simulink model "simproject2"  (R2022b)
settings: Solver=VariableStepAuto  StartTime=0.0  StopTime=Tsim  RelTol=1e-3
values from neighbouring files (symbols this model uses):
  Aroad = 5    [project2.m]
  Caf = 60000    [project2.m]
  Car = 60000    [project2.m]
  Iz = 2000    [project2.m]
  lambdaRoad = 100    [project2.m]
  lf = 1.1    [project2.m]
  lr = 1.3    [project2.m]
  m = 1050    [project2.m]
  Vx = 100/3.6    (= 27.7777777778)    [project2.m]
settings Model: Creator=Forough  LastModifiedBy=Forough

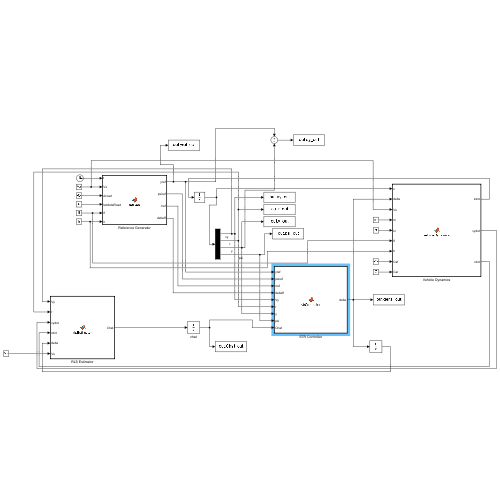
[thumbnail: Simulink's stored preview of the top-level diagram]
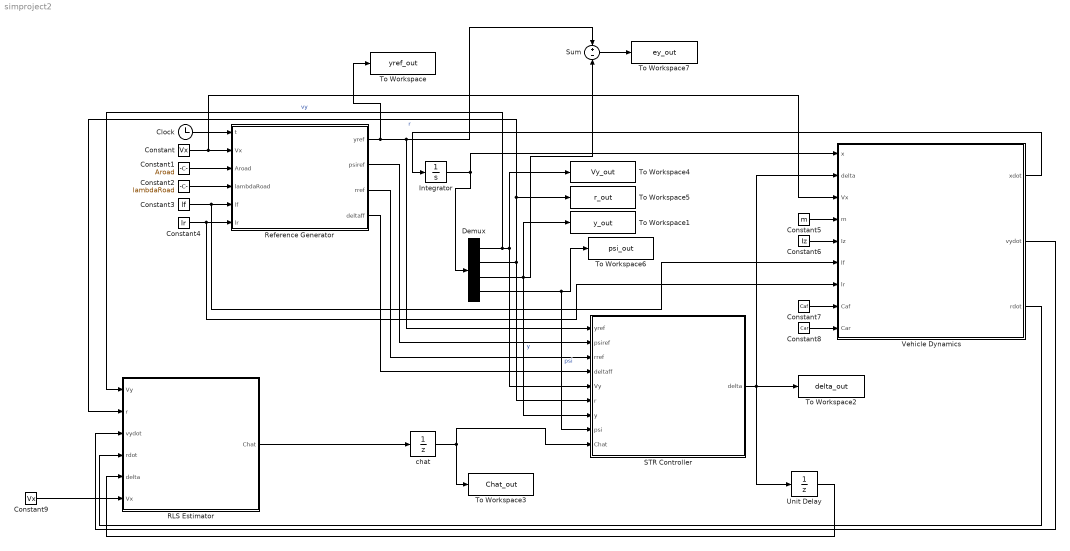
== system simproject2 ==
  Clock : Clock
  Constant : Constant  Value=Vx
  Constant1 : Constant  Value=Aroad
  Constant2 : Constant  Value=lambdaRoad
  Constant3 : Constant  Value=lf
  Constant4 : Constant  Value=lr
  Constant5 : Constant  Value=m
  Constant6 : Constant  Value=Iz
  Constant7 : Constant  Value=Caf
  Constant8 : Constant  Value=Car
  Constant9 : Constant  Value=Vx
  Demux : Demux
  Integrator : Integrator  InitialCondition=[0;0;0;0]
  RLS Estimator : MATLAB Function  TreatAsAtomicUnit=on
  Reference Generator : MATLAB Function  TreatAsAtomicUnit=on
  STR Controller : MATLAB Function  TreatAsAtomicUnit=on
  Sum : Sum  Inputs=+-
  To Workspace : ToWorkspace  VariableName=yref_out  SaveFormat=Timeseries  SampleTime=-1
  To Workspace1 : ToWorkspace  VariableName=y_out  SaveFormat=Timeseries  SampleTime=-1
  To Workspace2 : ToWorkspace  VariableName=delta_out  SaveFormat=Timeseries  SampleTime=-1
  To Workspace3 : ToWorkspace  VariableName=Chat_out  SaveFormat=Timeseries  SampleTime=-1
  To Workspace4 : ToWorkspace  VariableName=Vy_out  SaveFormat=Timeseries  SampleTime=-1
  To Workspace5 : ToWorkspace  VariableName=r_out  SaveFormat=Timeseries  SampleTime=-1
  To Workspace6 : ToWorkspace  VariableName=psi_out  SaveFormat=Timeseries  SampleTime=-1
  To Workspace7 : ToWorkspace  VariableName=ey_out  SaveFormat=Timeseries  SampleTime=-1
  Unit Delay : UnitDelay  SampleTime=0.001  HasFrameUpgradeWarning=on
  Vehicle Dynamics : MATLAB Function  TreatAsAtomicUnit=on
  chat : UnitDelay  InitialCondition=60000  SampleTime=0.001  HasFrameUpgradeWarning=on
  wires:
  Clock/1 -> Reference Generator/1(t)
  Integrator/1 -> Demux/1, Vehicle Dynamics/1(x)
  Vehicle Dynamics/1(xdot) -> Integrator/1
  Constant/1 -> Vehicle Dynamics/3(Vx), Reference Generator/2(Vx)
  Constant1/1 -> Reference Generator/3(Aroad)
  Constant2/1 -> Reference Generator/4(lambdaRoad)
  Constant3/1 -> Vehicle Dynamics/6(lf), Reference Generator/5(lf)
  Constant4/1 -> Vehicle Dynamics/7(lr), Reference Generator/6(lr)
  Reference Generator/1(yref) -> To Workspace/1, Sum/1, STR Controller/1(yref)
  Reference Generator/2(psiref) -> STR Controller/2(psiref)
  Reference Generator/3(rref) -> STR Controller/3(rref)
  Reference Generator/4(deltaff) -> STR Controller/4(deltaff)
  Demux/1 -> RLS Estimator/1(Vy), To Workspace4/1, STR Controller/5(Vy)  "vy"
  Demux/2 -> To Workspace5/1, RLS Estimator/2(r), STR Controller/6(r)  "r"
  Demux/3 -> Sum/2, To Workspace1/1, STR Controller/7(y)  "y"
  Demux/4 -> To Workspace6/1, STR Controller/8(psi)  "psi"
  RLS Estimator/1(Chat) -> chat/1
  STR Controller/1(delta) -> Unit Delay/1, To Workspace2/1, Vehicle Dynamics/2(delta)
  Unit Delay/1 -> RLS Estimator/5(delta)
  Vehicle Dynamics/2(vydot) -> RLS Estimator/3(vydot)
  Vehicle Dynamics/3(rdot) -> RLS Estimator/4(rdot)
  Constant5/1 -> Vehicle Dynamics/4(m)
  Constant6/1 -> Vehicle Dynamics/5(Iz)
  Constant7/1 -> Vehicle Dynamics/8(Caf)
  Constant8/1 -> Vehicle Dynamics/9(Car)
  chat/1 -> To Workspace3/1, STR Controller/9(Chat)
  Sum/1 -> To Workspace7/1
  Constant9/1 -> RLS Estimator/6(Vx)

== matlab function simproject2/Vehicle Dynamics ==
  data: x input; xdot output; delta input; Vx input; m input; Iz input; lf input; lr input; Caf input; Car input; vydot output; rdot output
function [xdot, vydot, rdot] = vehicleDynamics(x, delta, Vx, m, Iz, lf, lr, Caf, Car)

% States
Vy  = x(1);
r   = x(2);
y   = x(3);
psi = x(4);

% Lateral velocity dynamics
vydot = ...
    - ((2*Caf + 2*Car)/(m*Vx))*Vy ...
    - (Vx + (2*lf*Caf - 2*lr*Car)/(m*Vx))*r ...
    + (2*Caf/m)*delta;

% Yaw rate dynamics
rdot = ...
    - ((2*lf*Caf - 2*lr*Car)/(Iz*Vx))*Vy ...
    - ((2*lf^2*Caf + 2*lr^2*Car)/(Iz*Vx))*r ...
    + (2*lf*Caf/Iz)*delta;

% Global lateral position dynamics
ydot = Vy + Vx*psi;

% Yaw angle dynamics
psidot = r;

xdot = [vydot; rdot; ydot; psidot];

end

== matlab function simproject2/Reference Generator ==
  data: t input; yref output; Vx input; Aroad input; lambdaRoad input; lf input; lr input; psiref output; rref output; deltaff output
function [yref, psiref, rref, deltaff] = refGen(t, Vx, Aroad, lambdaRoad, lf, lr)

k = 2*pi/lambdaRoad;
x = Vx*t;

% Reference lateral position
yref = Aroad*sin(k*x);

% dy/dx
yp = Aroad*k*cos(k*x);

% d2y/dx2
ypp = -Aroad*k^2*sin(k*x);

% Reference yaw angle
psiref = atan(yp);

% Reference yaw rate
rref = (Vx*ypp)/(1 + yp^2);

% Curvature
kappa = ypp/(1 + yp^2)^(3/2);

% Feedforward steering
L = lf + lr;
deltaff = L*kappa;

end

== matlab function simproject2/RLS Estimator ==
  settings: updateMethod=DISCRETE
  data: Vy input; Chat output; r input; vydot input; rdot input; delta input; Vx input
function Chat = rlsEstimator(Vy, r, vydot, rdot, delta, Vx)

% Vehicle parameters
m  = 1050;
Iz = 2000;
lf = 1.1;
lr = 1.3;

% RLS parameters
lambda = 0.995;

persistent theta P

if isempty(theta)
    % Initial estimate intentionally selected lower than true value
    % to show convergence
    theta = 30000;
    P = 1e4;
end

% ---------- Input safety ----------
if ~isfinite(Vx) || abs(Vx) < 1
    Vx = 1;
end

if ~isfinite(Vy)
    Vy = 0;
end

if ~isfinite(r)
    r = 0;
end

if ~isfinite(vydot)
    vydot = 0;
end

if ~isfinite(rdot)
    rdot = 0;
end

if ~isfinite(delta)
    delta = 0;
end

% ---------- Protect persistent variables ----------
if ~isfinite(theta)
    theta = 30000;
end

if ~isfinite(P) || P <= 0 || P > 1e7
    P = 1e4;
end

% ==========================================================
% Regression equation 1 from lateral dynamics
% Y1 = phi1 * C_alpha
% ==========================================================

Y1 = m*(vydot + Vx*r);

phi1 = 2*delta ...
       - (2*(lf-lr)/Vx)*r ...
       - (4/Vx)*Vy;

% ==========================================================
% Regression equation 2 from yaw dynamics
% Y2 = phi2 * C_alpha
% ==========================================================

Y2 = Iz*rdot;

phi2 = 2*lf*delta ...
       - (2*(lf^2 + lr^2)/Vx)*r ...
       - (2*(lf-lr)/Vx)*Vy;

% Combine the two equations to improve estimation
Y = [Y1; Y2];
phi = [phi1; phi2];

% ---------- RLS update ----------
if all(isfinite(Y)) && all(isfinite(phi)) && norm(phi) > 1e-4 && norm(Y) < 1e8

    % Since theta is scalar, denominator is scalar
    den = lambda + phi' * P * phi;

    if isfinite(den) && den > 1e-9

        K = (P * phi) / den;   % 2x1 gain vector

        if all(isfinite(K))

            prediction_error = Y - phi * theta;

            if all(isfinite(prediction_error)) && norm(prediction_error) < 1e8

                theta_candidate = theta + K' * prediction_error;

                if isfinite(theta_candidate)

                    % Wider physical bounds so convergence is visible
                    if theta_candidate < 20000
                        theta_candidate = 20000;
                    elseif theta_candidate > 90000
                        theta_candidate = 90000;
                    end

                    % Moderate smoothing:
                    % larger alpha = faster visible convergence
                    alpha = 0.05;
                    theta = (1-alpha)*theta + alpha*theta_candidate;
                end
            end

            P_candidate = (P - K' * phi * P) / lambda;

            if isfinite(P_candidate) && P_candidate > 1e-6 && P_candidate < 1e7
                P = P_candidate;
            else
                P = 1e4;
            end
        end
    end
end

% ---------- Final output protection ----------
if ~isfinite(theta)
    theta = 30000;
end

% Final physical limits
if theta < 20000
    theta = 20000;
elseif theta > 90000
    theta = 90000;
end

Chat = theta;

end

== matlab function simproject2/STR Controller ==
  settings: updateMethod=DISCRETE
  data: yref input; psiref input; rref input; deltaff input; Vy input; delta output; r input; y input; psi input; Chat input
function delta = strController(yref, psiref, rref, deltaff, Vy, r, y, psi, Chat)

% ==========================================================
% Indirect STR / RST Controller for lateral path tracking
%
% The external RLS estimator provides Chat, which is the online
% estimate of the tire cornering stiffness C_alpha.
%
% In this controller, Chat is used to adapt the effective input
% gain of the identified error model. Since the steering-to-lateral
% response depends strongly on tire cornering stiffness, the B
% polynomial of the ARX error model is scaled using Chat/Cnom.
%
% Error definition:
% e(k) = y(k) - y_ref(k)
%
% Identified model:
% A(q^-1)e(k) = q^-1 B(q^-1)u_fb(k)
%
% RST control law:
% R(q^-1)u_fb(k) = -S(q^-1)e(k)
%
% Final steering:
% delta(k) = delta_ff(k) + u_fb(k) + damping terms
% ==========================================================

%% ==========================================================
% Sampling and update rate
% ==========================================================

Ts_sim = 0.001;     % Simulation sample time (s)
Tc     = 0.02;      % Controller update time (s)
Nhold  = round(Tc/Ts_sim);

%% ==========================================================
% Nominal parameters and limits
% ==========================================================

Cnom = 60000;       % Nominal cornering stiffness (N/rad)
Cmin = 20000;       % Lower physical bound for estimated stiffness
Cmax = 90000;       % Upper physical bound for estimated stiffness

deltaMax = 0.25;    % Steering saturation limit (rad)

%% ==========================================================
% Persistent variables
% ==========================================================

persistent cnt delta_hold

persistent e1 e2
persistent u1 u2

persistent theta P

persistent satCounter

if isempty(cnt)

    cnt = 0;
    delta_hold = 0;

    e1 = 0;
    e2 = 0;

    u1 = 0;
    u2 = 0;

    % Initial ARX model:
    % e(k) = -a1 e(k-1) - a2 e(k-2) + b0 u(k-1) + b1 u(k-2)
    %
    % A(q^-1) = 1 + a1 q^-1 + a2 q^-2
    % B(q^-1) = b0 + b1 q^-1

    theta = [-1.65; 0.70; 0.015; 0.004];

    P = 100*eye(4);

    satCounter = 0;
end

%% ==========================================================
% Hold control signal between controller updates
% ==========================================================

cnt = cnt + 1;

if cnt < Nhold
    delta = delta_hold;
    return;
end

cnt = 0;

%% ==========================================================
% Safety checks for inputs
% ==========================================================

if ~isfinite(yref)
    yref = 0;
end

if ~isfinite(y)
    y = 0;
end

if ~isfinite(deltaff)
    deltaff = 0;
end

if ~isfinite(Chat)
    Chat = Cnom;
end

if Chat < Cmin
    Chat = Cmin;
elseif Chat > Cmax
    Chat = Cmax;
end

if ~isfinite(Vy)
    Vy = 0;
end

if ~isfinite(r)
    r = 0;
end

if ~isfinite(psi)
    psi = 0;
end

if ~isfinite(psiref)
    psiref = 0;
end

if ~isfinite(rref)
    rref = 0;
end

%% ==========================================================
% 1) Define lateral tracking error
% ==========================================================

e = y - yref;

if ~isfinite(e)
    e = 0;
end

%% ==========================================================
% 2) Online ARX identification of lateral error dynamics
%
% e(k) = phi^T theta
%
% theta = [a1; a2; b0; b1]
% phi   = [-e(k-1); -e(k-2); u(k-1); u(k-2)]
% ==========================================================

lambda = 0.995;

phi = [-e1; -e2; u1; u2];

if all(isfinite(phi)) && isfinite(e) && norm(phi) > 1e-6

    den = lambda + phi.'*P*phi;

    if isfinite(den) && den > 1e-9

        Krls = P*phi/den;
        eps  = e - phi.'*theta;

        if all(isfinite(Krls)) && isfinite(eps)

            theta_raw = theta + Krls*eps;

            a1n = theta_raw(1);
            a2n = theta_raw(2);
            b0n = theta_raw(3);
            b1n = theta_raw(4);

            % Keep A polynomial inside a conservative stable range
            if a1n < -1.9
                a1n = -1.9;
            elseif a1n > 1.9
                a1n = 1.9;
            end

            if a2n < 0.05
                a2n = 0.05;
            elseif a2n > 0.95
                a2n = 0.95;
            end

            % Keep B polynomial physically meaningful
            if b0n < 1e-4
                b0n = 1e-4;
            elseif b0n > 0.2
                b0n = 0.2;
            end

            if b1n < -0.2
                b1n = -0.2;
            elseif b1n > 0.2
                b1n = 0.2;
            end

            theta_candidate = [a1n; a2n; b0n; b1n];

            % Smooth parameter update to avoid abrupt controller changes
            alpha = 0.02;
            theta = (1-alpha)*theta + alpha*theta_candidate;

            Pnew = (P - Krls*phi.'*P)/lambda;

            if all(isfinite(Pnew(:)))
                P = Pnew;
            else
                P = 100*eye(4);
            end
        end
    end
end

a1 = theta(1);
a2 = theta(2);
b0 = theta(3);
b1 = theta(4);

%% ==========================================================
% 3) Use estimated tire stiffness in the STR design
%
% The steering effectiveness depends on tire stiffness.
% Therefore, the B polynomial is scaled by Chat/Cnom.
% If Chat decreases, the effective steering gain decreases.
% If Chat increases, the effective steering gain increases.
% ==========================================================

Cscale = Chat / Cnom;

if Cscale < 0.4
    Cscale = 0.4;
elseif Cscale > 1.5
    Cscale = 1.5;
end

b0_eff = b0 * Cscale;
b1_eff = b1 * Cscale;

% Protection against too small input gain
if abs(b0_eff) < 1e-5
    b0_eff = sign(b0_eff + 1e-12)*1e-5;
end

%% ==========================================================
% 4) Desired closed-loop polynomial
%
% Ac(q^-1) = (1 - pc1 q^-1)(1 - pc2 q^-1)(1 - po q^-1)
% ==========================================================

pc1 = 0.82;
pc2 = 0.78;
po  = 0.55;

Ac1 = -(pc1 + pc2 + po);
Ac2 = pc1*pc2 + pc1*po + pc2*po;
Ac3 = -pc1*pc2*po;

%% ==========================================================
% 5) Solve Diophantine equation
%
% A(q^-1)R(q^-1) + q^-1 B(q^-1)S(q^-1) = Ac(q^-1)
%
% A = 1 + a1 q^-1 + a2 q^-2
% B = b0_eff + b1_eff q^-1
% R = 1 + r1 q^-1
% S = s0 + s1 q^-1
% ==========================================================

M = [1,  b0_eff,  0;
     a1, b1_eff,  b0_eff;
     a2, 0,       b1_eff];

rhs = [Ac1 - a1;
       Ac2 - a2;
       Ac3];

useBackup = false;

if ~all(isfinite(M(:))) || ~all(isfinite(rhs(:)))
    useBackup = true;
end

if ~useBackup
    if rcond(M) < 1e-8
        useBackup = true;
    end
end

if ~useBackup
    sol = M\rhs;
    rr1 = sol(1);
    s0  = sol(2);
    s1  = sol(3);
else
    rr1 = 0.0;
    s0  = 0.015;
    s1  = 0.0;
end

if ~isfinite(rr1)
    rr1 = 0;
end

if ~isfinite(s0)
    s0 = 0.015;
end

if ~isfinite(s1)
    s1 = 0;
end

% Conservative limits for controller coefficients
if rr1 > 1.2
    rr1 = 1.2;
elseif rr1 < -1.2
    rr1 = -1.2;
end

if s0 > 0.08
    s0 = 0.08;
elseif s0 < -0.08
    s0 = -0.08;
end

if s1 > 0.08
    s1 = 0.08;
elseif s1 < -0.08
    s1 = -0.08;
end

%% ==========================================================
% 6) RST regulation law
%
% R u_fb = -S e
%
% (1 + rr1 q^-1)u(k) = -s0 e(k) - s1 e(k-1)
%
% u(k) = -rr1 u(k-1) - s0 e(k) - s1 e(k-1)
% ==========================================================

u_rst = -rr1*u1 - s0*e - s1*e1;

%% ==========================================================
% 7) Additional damping terms
%
% These terms improve yaw stability and reduce oscillations.
% ==========================================================

Kpsi = 0.25;
Kr   = 0.035;
Kvy  = 0.006;

u_damp = Kpsi*(psiref - psi) + Kr*(rref - r) - Kvy*Vy;

%% ==========================================================
% 8) Final steering command
% ==========================================================

delta_unsat = deltaff + u_rst + u_damp;

if delta_unsat > deltaMax
    delta_new = deltaMax;
elseif delta_unsat < -deltaMax
    delta_new = -deltaMax;
else
    delta_new = delta_unsat;
end

if ~isfinite(delta_new)
    delta_new = 0;
end

%% ==========================================================
% 9) Anti-sticking protection
%
% If the controller remains near saturation for too long,
% the steering command is slightly reduced.
% ==========================================================

if abs(delta_new) >= 0.249
    satCounter = satCounter + 1;
else
    satCounter = 0;
end

if satCounter > 20
    delta_new = 0.7*delta_new;
    satCounter = 0;
end

%% ==========================================================
% 10) Update histories
% ==========================================================

e2 = e1;
e1 = e;

u2 = u1;
u1 = delta_new - deltaff;

delta_hold = delta_new;
delta = delta_hold;

end
